simulink model "Elem9_L5_NL4_modified"  (R2023a)
settings: Solver=ode4  StartTime=0.0  StopTime=10.0  RelTol=1e-3
values from neighbouring files (symbols this model uses):
  element : value not decoded    [Elem9_L5_NL4.sldd]
  model : value not decoded    [Elem9_L5_NL4.sldd]
settings Model: DataDictionary=Elem9_L5_NL4.sldd  Creator=glenn  LastModifiedBy=glenn

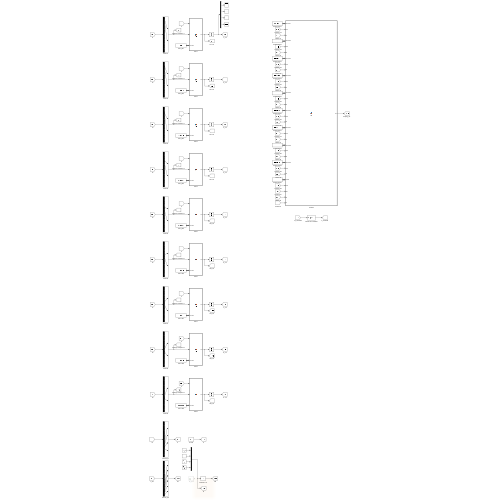
[thumbnail: Simulink's stored preview of the top-level diagram]
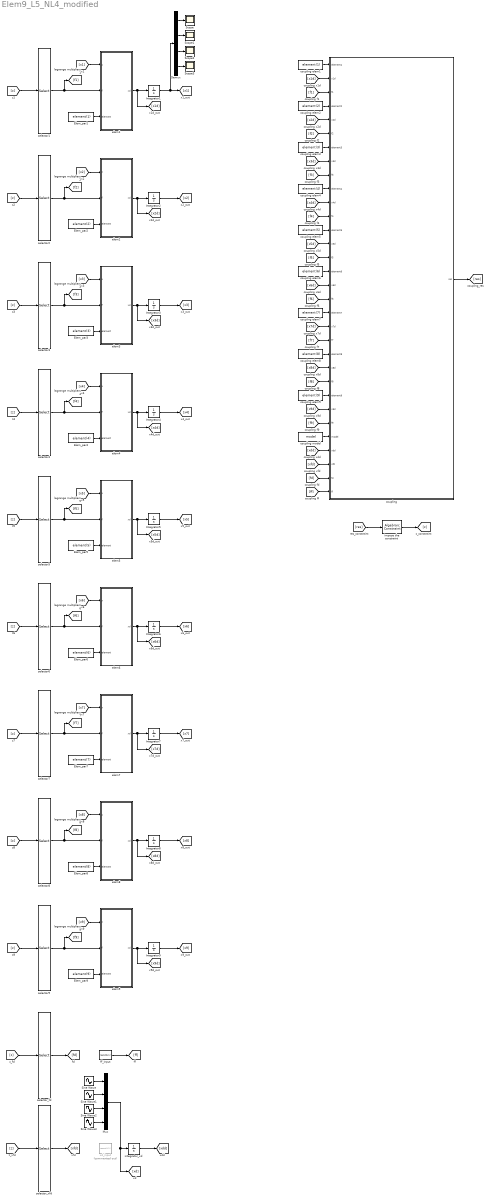
== system Elem9_L5_NL4_modified ==
  Demux : Demux
  Elem_par1 : Constant  Value=element(1)  OutDataTypeStr=Bus: ePar1
  Elem_par2 : Constant  Value=element(2)  OutDataTypeStr=Bus: ePar2
  Elem_par3 : Constant  Value=element(3)  OutDataTypeStr=Bus: ePar3
  Elem_par4 : Constant  Value=element(4)  OutDataTypeStr=Bus: ePar4
  Elem_par5 : Constant  Value=element(5)  OutDataTypeStr=Bus: ePar5
  Elem_par6 : Constant  Value=element(6)  OutDataTypeStr=Bus: ePar6
  Elem_par7 : Constant  Value=element(7)  OutDataTypeStr=Bus: ePar7
  Elem_par8 : Constant  Value=element(8)  OutDataTypeStr=Bus: ePar8
  Elem_par9 : Constant  Value=element(9)  OutDataTypeStr=Bus: ePar9
  Integrator{1..3,8..9} (5 alike) : Integrator  InitialCondition=zeros(4,1)
  Integrator{4..7} (4 alike) : Integrator  InitialCondition=zeros(5,1)
  Mux : Mux
  Scope{,1..3} (4 alike) : Scope
  Sine Wave{,1..3} (4 alike) : Sin  SampleTime=0
  coupling : MATLAB Function  TreatAsAtomicUnit=on
  coupling elem1 : Constant  Value=element(1)  OutDataTypeStr=Bus: ePar1
  coupling elem2 : Constant  Value=element(2)  OutDataTypeStr=Bus: ePar2
  coupling elem3 : Constant  Value=element(3)  OutDataTypeStr=Bus: ePar3
  coupling elem4 : Constant  Value=element(4)  OutDataTypeStr=Bus: ePar4
  coupling elem5 : Constant  Value=element(5)  OutDataTypeStr=Bus: ePar5
  coupling elem6 : Constant  Value=element(6)  OutDataTypeStr=Bus: ePar6
  coupling elem7 : Constant  Value=element(7)  OutDataTypeStr=Bus: ePar7
  coupling elem8 : Constant  Value=element(8)  OutDataTypeStr=Bus: ePar8
  coupling elem9 : Constant  Value=element(9)  OutDataTypeStr=Bus: ePar9
  coupling model : Constant  Value=model  OutDataTypeStr=Bus: mPar
  elem1 : MATLAB Function  TreatAsAtomicUnit=on
  elem2 : MATLAB Function  TreatAsAtomicUnit=on
  elem3 : MATLAB Function  TreatAsAtomicUnit=on
  elem4 : MATLAB Function  TreatAsAtomicUnit=on
  elem5 : MATLAB Function  TreatAsAtomicUnit=on
  elem6 : MATLAB Function  TreatAsAtomicUnit=on
  elem7 : MATLAB Function  TreatAsAtomicUnit=on
  elem8 : MATLAB Function  TreatAsAtomicUnit=on
  elem9 : MATLAB Function  TreatAsAtomicUnit=on
  ff_input : Constant  Value=zeros(6,1)
  impose the constraint : AlgebraicConstraint
  integrator_xd : Integrator  InitialCondition=zeros(4,1)
  selector1 : Selector  InputPortWidth=28  IndexOptions=Index vector (dialog)  Indices="[1  2]"  OutputSizes=1
  selector2 : Selector  InputPortWidth=28  IndexOptions=Index vector (dialog)  Indices="[3  4]"  OutputSizes=1
  selector3 : Selector  InputPortWidth=28  IndexOptions=Index vector (dialog)  Indices="[5  6]"  OutputSizes=1
  selector4 : Selector  InputPortWidth=28  IndexOptions=Index vector (dialog)  Indices="[7  8]"  OutputSizes=1
  selector5 : Selector  InputPortWidth=28  IndexOptions=Index vector (dialog)  Indices="[9  10]"  OutputSizes=1
  selector6 : Selector  InputPortWidth=28  IndexOptions=Index vector (dialog)  Indices="[11  12]"  OutputSizes=1
  selector7 : Selector  InputPortWidth=28  IndexOptions=Index vector (dialog)  Indices="[13  14]"  OutputSizes=1
  selector8 : Selector  InputPortWidth=28  IndexOptions=Index vector (dialog)  Indices="[15  16]"  OutputSizes=1
  selector9 : Selector  InputPortWidth=28  IndexOptions=Index vector (dialog)  Indices="[17  18]"  OutputSizes=1
  selector_fd : Selector  InputPortWidth=28  IndexOptions=Index vector (dialog)  Indices="[19  20  21  22]"  OutputSizes=1
  selector_xfd : Selector  InputPortWidth=28  IndexOptions=Index vector (dialog)  Indices="[23  24  25  26  27  28]"  OutputSizes=1
  xd_input : Constant  Commented=on  Value=zeros(4,1)
  wires:
  [x1] -> elem1/1(x)
  selector1/1 -> elem1/2(f), [f1]
  [z] -> selector1/1
  Elem_par1/1 -> elem1/3(element)
  elem1/1(xd) -> Integrator1/1, [x1d]
  Integrator1/1 -> Demux/1, [x1]
  coupling elem1/1 -> coupling/1(element1)
  [x1d] -> coupling/2(x1d)
  [f1] -> coupling/3(f1)
  [x2] -> elem2/1(x)
  selector2/1 -> elem2/2(f), [f2]
  [z] -> selector2/1
  Elem_par2/1 -> elem2/3(element)
  elem2/1(xd) -> Integrator2/1, [x2d]
  Integrator2/1 -> [x2]
  coupling elem2/1 -> coupling/4(element2)
  [x2d] -> coupling/5(x2d)
  [f2] -> coupling/6(f2)
  [x3] -> elem3/1(x)
  selector3/1 -> elem3/2(f), [f3]
  [z] -> selector3/1
  Elem_par3/1 -> elem3/3(element)
  elem3/1(xd) -> Integrator3/1, [x3d]
  Integrator3/1 -> [x3]
  coupling elem3/1 -> coupling/7(element3)
  [x3d] -> coupling/8(x3d)
  [f3] -> coupling/9(f3)
  [x4] -> elem4/1(x)
  selector4/1 -> elem4/2(f), [f4]
  [z] -> selector4/1
  Elem_par4/1 -> elem4/3(element)
  elem4/1(xd) -> Integrator4/1, [x4d]
  Integrator4/1 -> [x4]
  coupling elem4/1 -> coupling/10(element4)
  [x4d] -> coupling/11(x4d)
  [f4] -> coupling/12(f4)
  [x5] -> elem5/1(x)
  selector5/1 -> elem5/2(f), [f5]
  [z] -> selector5/1
  Elem_par5/1 -> elem5/3(element)
  elem5/1(xd) -> Integrator5/1, [x5d]
  Integrator5/1 -> [x5]
  coupling elem5/1 -> coupling/13(element5)
  [x5d] -> coupling/14(x5d)
  [f5] -> coupling/15(f5)
  [x6] -> elem6/1(x)
  selector6/1 -> elem6/2(f), [f6]
  [z] -> selector6/1
  Elem_par6/1 -> elem6/3(element)
  elem6/1(xd) -> Integrator6/1, [x6d]
  Integrator6/1 -> [x6]
  coupling elem6/1 -> coupling/16(element6)
  [x6d] -> coupling/17(x6d)
  [f6] -> coupling/18(f6)
  [x7] -> elem7/1(x)
  selector7/1 -> elem7/2(f), [f7]
  [z] -> selector7/1
  Elem_par7/1 -> elem7/3(element)
  elem7/1(xd) -> Integrator7/1, [x7d]
  Integrator7/1 -> [x7]
  coupling elem7/1 -> coupling/19(element7)
  [x7d] -> coupling/20(x7d)
  [f7] -> coupling/21(f7)
  [x8] -> elem8/1(x)
  selector8/1 -> elem8/2(f), [f8]
  [z] -> selector8/1
  Elem_par8/1 -> elem8/3(element)
  elem8/1(xd) -> Integrator8/1, [x8d]
  Integrator8/1 -> [x8]
  coupling elem8/1 -> coupling/22(element8)
  [x8d] -> coupling/23(x8d)
  [f8] -> coupling/24(f8)
  [x9] -> elem9/1(x)
  selector9/1 -> elem9/2(f), [f9]
  [z] -> selector9/1
  Elem_par9/1 -> elem9/3(element)
  elem9/1(xd) -> Integrator9/1, [x9d]
  Integrator9/1 -> [x9]
  coupling elem9/1 -> coupling/25(element9)
  [x9d] -> coupling/26(x9d)
  [f9] -> coupling/27(f9)
  coupling model/1 -> coupling/28(model)
  [xdd] -> coupling/29(xdd)
  [xfd] -> coupling/30(xfd)
  [fd] -> coupling/31(fd)
  [ff] -> coupling/32(ff)
  coupling/1(res) -> [res]
  [z] -> selector_fd/1
  [z] -> selector_xfd/1
  selector_fd/1 -> [fd]
  selector_xfd/1 -> [xfd]
  ff_input/1 -> [ff]
  integrator_xd/1 -> [xdd]
  [res] -> impose the constraint/1
  impose the constraint/1 -> [z]
  Demux/1 -> Scope/1
  Demux/2 -> Scope1/1
  Demux/3 -> Scope2/1
  Demux/4 -> Scope3/1
  Sine Wave/1 -> Mux/1
  Sine Wave3/1 -> Mux/4
  Sine Wave2/1 -> Mux/3
  Sine Wave1/1 -> Mux/2
  Mux/1 -> [xd], integrator_xd/1

== matlab function Elem9_L5_NL4_modified/elem8 ==
  data: x input; xd output; f input; element input
function xd = fcn(x,f,element)

xd = element.M \ (element.B*f - evalR(x, element));

end

function R = evalR(x, element)

R = pierR_linear(x, element);

end

== matlab function Elem9_L5_NL4_modified/elem9 ==
  data: x input; xd output; f input; element input
function xd = fcn(x,f,element)

xd = element.M \ (element.B*f - evalR(x, element));

end

function R = evalR(x, element)

R = pierR_linear(x, element);

end

== matlab function Elem9_L5_NL4_modified/coupling ==
  data: element1 input; res output; x1d input; f1 input; element2 input; x2d input; f2 input; element3 input; x3d input; f3 input; element4 input; x4d input; f4 input; element5 input; x5d input; f5 input; element6 input; x6d input; f6 input; element7 input; x7d input; f7 input; element8 input; x8d input; f8 input; element9 input; x9d input; f9 input; model input; xdd input; xfd input; fd input; ff input
function res = fcn(element1,x1d,f1,element2,x2d,f2,element3,x3d,f3,element4,x4d,f4,element5,x5d,f5,element6,x6d,f6,element7,x7d,f7,element8,x8d,f8,element9,x9d,f9,model,xdd,xfd,fd,ff)

% Equilibrium
epsilon_B = element1.Bbar * f1 + element2.Bbar * f2 + element3.Bbar * f3 + element4.Bbar * f4 + element5.Bbar * f5 + element6.Bbar * f6 + element7.Bbar * f7 + element8.Bbar * f8 + element9.Bbar * f9 + model.Bbar_f * ff + model.Bbar_d * fd;

% Compatibility
epsilon_G = [
element1.G_f * x1d + element1.Gbar_f * xfd ;
element2.G_f * x2d + element2.Gbar_f * xfd ;
element3.G_f * x3d + element3.Gbar_f * xfd ;
[element4.G_f; element4.G_d] * x4d + blkdiag(element4.Gbar_f, element4.Gbar_d) * [xfd; xdd] ;
element5.G_f * x5d + element5.Gbar_f * xfd ;
element6.G_f * x6d + element6.Gbar_f * xfd ;
[element7.G_f; element7.G_d] * x7d + blkdiag(element7.Gbar_f, element7.Gbar_d) * [xfd; xdd] ;
[element8.G_f; element8.G_d] * x8d + blkdiag(element8.Gbar_f, element8.Gbar_d) * [xfd; xdd] ;
[element9.G_f; element9.G_d] * x9d + blkdiag(element9.Gbar_f, element9.Gbar_d) * [xfd; xdd] ;
];

% Residuals
res = [epsilon_B; epsilon_G];

end

== matlab function Elem9_L5_NL4_modified/elem2 ==
  data: x input; xd output; f input; element input
function xd = fcn(x,f,element)

xd = element.M \ (element.B*f - evalR(x, element));

end

function R = evalR(x, element)

R = pierR_linear(x, element);

end

== matlab function Elem9_L5_NL4_modified/elem1 ==
  data: x input; xd output; f input; element input
function xd = fcn(x,f,element)

xd = element.M \ (element.B*f - evalR(x, element));

end

function R = evalR(x, element)

R = pierR_linear(x, element);

end

== matlab function Elem9_L5_NL4_modified/elem3 ==
  data: x input; xd output; f input; element input
function xd = fcn(x,f,element)

xd = element.M \ (element.B*f - evalR(x, element));

end

function R = evalR(x, element)

R = pierR_linear(x, element);

end

== matlab function Elem9_L5_NL4_modified/elem4 ==
  data: x input; xd output; f input; element input
function xd = fcn(x,f,element)

xd = element.M \ (element.B*f - evalR(x, element));

end

function R = evalR(x, element)

R = pierR_mostaghel(x, element);

end

== matlab function Elem9_L5_NL4_modified/elem5 ==
  data: x input; xd output; f input; element input
function xd = fcn(x,f,element)

xd = element.M \ (element.B*f - evalR(x, element));

end

function R = evalR(x, element)

R = pierR_mostaghel(x, element);

end

== matlab function Elem9_L5_NL4_modified/elem6 ==
  data: x input; xd output; f input; element input
function xd = fcn(x,f,element)

xd = element.M \ (element.B*f - evalR(x, element));

end

function R = evalR(x, element)

R = pierR_mostaghel(x, element);

end

== matlab function Elem9_L5_NL4_modified/elem7 ==
  data: x input; xd output; f input; element input
function xd = fcn(x,f,element)

xd = element.M \ (element.B*f - evalR(x, element));

end

function R = evalR(x, element)

R = pierR_mostaghel(x, element);

end
